simulink model "taketwo_v2"  (R2025a)
settings: Solver=FixedStepAuto  StartTime=0.0  StopTime=100  FixedStep=0.05  RelTol=1e-3
libraries: robotlib x7

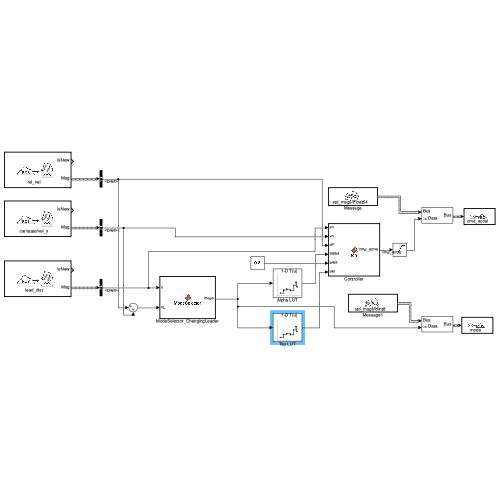
[thumbnail: Simulink's stored preview of the top-level diagram]
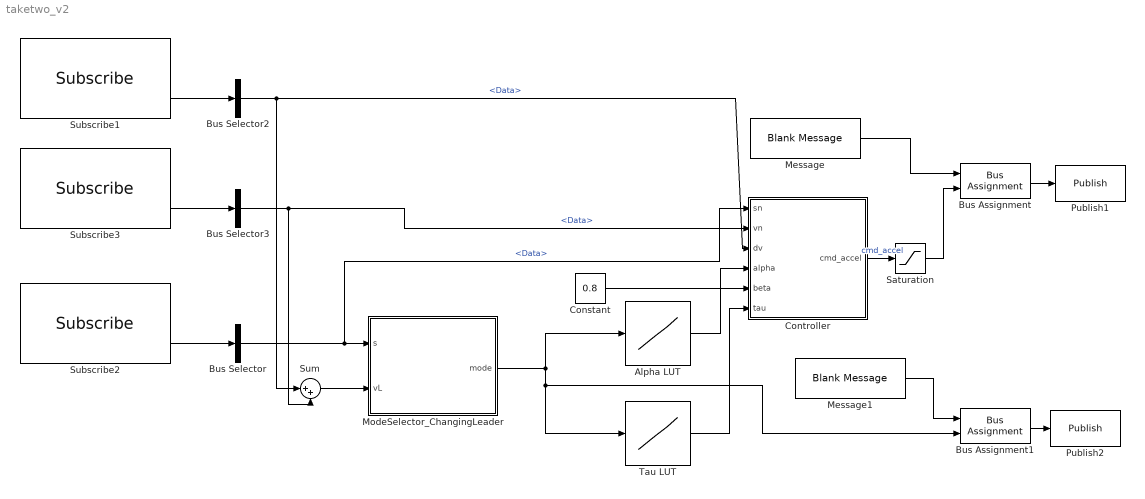
== system taketwo_v2 ==
  Alpha LUT : Lookup_n-D  NumberOfTableDimensions=1  BreakpointsForDimension1=[0 1 2 3]  Table=[0.75 0.75 1.0 0.25]  InterpMethod=Nearest  InternalRulePriority=Speed  RndMeth=Simplest
  Bus Assignment : BusAssignment  AssignedSignals=Data
  Bus Assignment1 : BusAssignment  AssignedSignals=Data
  Bus Selector : BusSelector  OutputSignals=Data
  Bus Selector2 : BusSelector  OutputSignals=Data
  Bus Selector3 : BusSelector  OutputSignals=Data
  Constant : Constant  Value=0.8
  Controller : MATLAB Function  TreatAsAtomicUnit=on
  Message : robotlib/Blank Message  messageClass=Message  entityType=std_msgs/Float64  messageType=std_msgs/Float64  SampleTime=inf  legacyBusStruct=off
  Message1 : robotlib/Blank Message  messageClass=Message  entityType=std_msgs/UInt8  messageType=std_msgs/UInt8  SampleTime=inf  legacyBusStruct=off
  ModeSelector_ChangingLeader : MATLAB Function  TreatAsAtomicUnit=on
  Publish1 : robotlib/Publish  topicSource=Specify your own  topic=cmd_accel  messageType=std_msgs/Float64  legacyBusStruct=off  messageQueueLength=1
  Publish2 : robotlib/Publish  topicSource=Specify your own  topic=mode  messageType=std_msgs/UInt8  legacyBusStruct=off  messageQueueLength=1
  Saturation : Saturate  UpperLimit=1.5  LowerLimit=-3.0
  Subscribe1 : robotlib/Subscribe  topicSource=Specify your own  topic=rel_vel  messageType=std_msgs/Float64  SampleTime=0.05  legacyBusStruct=off  messageQueueLength=1
  Subscribe2 : robotlib/Subscribe  topicSource=Specify your own  topic=lead_dist  messageType=std_msgs/Float64  SampleTime=0.05  legacyBusStruct=off  messageQueueLength=1
  Subscribe3 : robotlib/Subscribe  topicSource=Specify your own  topic=car/state/vel_x  messageType=std_msgs/Float64  SampleTime=0.05  legacyBusStruct=off  messageQueueLength=1
  Sum : Sum  Inputs=|++
  Tau LUT : Lookup_n-D  NumberOfTableDimensions=1  BreakpointsForDimension1=[0 1 2 3]  Table=[0.75 1.0 0.5 2.0]  InterpMethod=Nearest  InternalRulePriority=Speed  RndMeth=Simplest
  wires:
  Tau LUT/1 -> Controller/6(tau)
  ModeSelector_ChangingLeader/1(mode) -> Tau LUT/1, Bus Assignment1/2, Alpha LUT/1
  Constant/1 -> Controller/5(beta)
  Alpha LUT/1 -> Controller/4(alpha)
  Bus Selector/1 -> Controller/1(sn), ModeSelector_ChangingLeader/1(s)  "<Data>"
  Bus Selector3/1 -> Controller/2(vn), Sum/2  "<Data>"
  Bus Selector2/1 -> Controller/3(dv), Sum/1  "<Data>"
  Sum/1 -> ModeSelector_ChangingLeader/2(vL)
  Controller/1(cmd_accel) -> Saturation/1  "cmd_accel"
  Saturation/1 -> Bus Assignment/2
  Subscribe1/2 -> Bus Selector2/1
  Subscribe3/2 -> Bus Selector3/1
  Subscribe2/2 -> Bus Selector/1
  Message/1 -> Bus Assignment/1
  Message1/1 -> Bus Assignment1/1
  Bus Assignment1/1 -> Publish2/1
  Bus Assignment/1 -> Publish1/1

== matlab function taketwo_v2/Controller ==
function cmd_accel = fcn(sn, vn, dv, alpha, beta, tau)
% sn   : geometric gap (lead back - ego front) [m]
% vn   : ego speed [m/s]
% dv   : v_lead - v_ego [m/s]   (NEG when ego is faster)

    % ---- force scalars in case any input arrives as a vector ----
    sn    = double(sn(1));
    vn    = double(vn(1));
    dv    = double(dv(1));
    alpha = double(alpha(1));
    beta  = double(beta(1));
    tau   = double(tau(1));

    % --- constants ---
    s_min = 20.0;     % standstill buffer [m]
    s_far = 150.0;    % use cruise control when gap > this [m]
    v_des = 20.0;    % desired cruise speed [m/s]
    a_min = -3.0;    % max braking  [m/s^2]
    a_max =  1.5;    % max accel    [m/s^2]

    % predeclare to fix output dimension
    a = 0.0;

    if sn > s_far
        % Far from leader: simple speed hold
        a = beta .* (v_des - vn);
    else
        % Within 150 m: time-gap + relative-velocity PD
        sn_eff = max(sn - s_min, 0.0);
        a = alpha .* (sn_eff - tau .* vn) + beta .* dv;

        % Emergency rule: inside buffer and still closing -> full brake
        if sn <= s_min && dv < 0
            a = a_min;
        end
    end

    % Clamp to actuator limits
    cmd_accel = min(max(a, a_min), a_max);
end

== matlab function taketwo_v2/ModeSelector_ChangingLeader ==
  settings: updateMethod=DISCRETE
function mode = ModeSelector(s, vL)
% 1 no leader, 2 collecting, 3 smooth, 4 erratic
%#codegen

% ---------- Tunables ----------
Ts               = 0.05;     % [s]
S_NOLEADER_IN    = 140.0;    % [m] enter-leader-present threshold (lower)
S_NOLEADER_OUT   = 160.0;    % [m] exit-leader-present threshold (higher)
COLLECT_SECS     = 15.0;     % [s]
S_JUMP_THR       = 15.0;     % [m]
EWMA_TAU         = 3.0;      % [s]
SIGMA_LOW        = 0.50;     % [m/s]
SIGMA_HIGH       = 0.80;     % [m/s]
SIGMA_DEBOUNCE   = 0.5;      % [s] must be consistently above/below to switch 3<->4
MODE_DWELL_SECS  = 2.0;      % [s] minimum time to hold a mode before switching
% --------------------------------

persistent inited prev_s leader_present collect_cnt mu var last_mode ...
           dwell_ctr sigma_hi_ctr sigma_lo_ctr
if isempty(inited)
    inited        = true;
    prev_s        = s;
    leader_present= (s <= S_NOLEADER_IN);
    collect_cnt   = int32( leader_present * round(COLLECT_SECS / Ts) );
    mu            = vL; var = 0.0;
    last_mode     = uint8(1);
    dwell_ctr     = int32( round(MODE_DWELL_SECS / Ts) );  % start “already dwelled”
    sigma_hi_ctr  = int32(0);
    sigma_lo_ctr  = int32(0);
end

% Distance hysteresis for leader presence
if  leader_present && (s >= S_NOLEADER_OUT), leader_present = false; end
if ~leader_present && (s <= S_NOLEADER_IN),  leader_present = true;  end

% Warm-up restarts
ds = s - prev_s;
if leader_present && ~ (prev_s <= S_NOLEADER_IN)
    collect_cnt = int32(round(COLLECT_SECS / Ts)); mu = vL; var = 0.0;
end
if abs(ds) >= S_JUMP_THR
    collect_cnt = int32(round(COLLECT_SECS / Ts)); mu = vL; var = 0.0;
end

% EWMA (only when leader present)
alpha = Ts / max(EWMA_TAU, Ts); if alpha > 1, alpha = 1; end
if leader_present
    mu  = (1 - alpha)*mu + alpha*vL;
    d   = vL - mu;
    var = (1 - alpha)*(var + alpha*d*d);
else
    mu = vL; var = 0.0;
end
sigma = sqrt(max(var,0.0));

% Sigma debounce counters (require consistency for SIGMA_DEBOUNCE)
need = int32( max(1, round(SIGMA_DEBOUNCE / Ts)) );
if sigma >= SIGMA_HIGH,  sigma_hi_ctr = min(need, sigma_hi_ctr+1); else, sigma_hi_ctr = int32(0); end
if sigma <= SIGMA_LOW,   sigma_lo_ctr = min(need, sigma_lo_ctr+1); else, sigma_lo_ctr = int32(0); end

% Dwell time counter
if dwell_ctr < need, dwell_ctr = dwell_ctr + 1; end

% ----- Mode decision with dwell/debounce/hysteresis -----
if ~leader_present
    mode = uint8(1);                       % cruise/no leader
    dwell_ctr = int32(0);
elseif collect_cnt > 0
    collect_cnt = collect_cnt - 1;
    mode = uint8(2);                       % warm-up
    dwell_ctr = int32(0);
else
    % Only allow 3<->4 switch when dwell satisfied AND debounce holds
    if last_mode == uint8(4)
        if (dwell_ctr >= need) && (sigma_lo_ctr >= need)
            mode = uint8(3);
            dwell_ctr = int32(0);
        else
            mode = uint8(4);
        end
    else % last_mode is 1/2/3 (treat 1/2 as 3 for hysteresis after warm-up)
        if last_mode == uint8(1) || last_mode == uint8(2), last_mode = uint8(3); end
        if (dwell_ctr >= need) && (sigma_hi_ctr >= need)
            mode = uint8(4);
            dwell_ctr = int32(0);
        else
            mode = uint8(3);
        end
    end
end

% Bookkeeping
last_mode = mode;
prev_s    = s;
